simulink model "LQRPressureControl_simulation"  (R2020b)
settings: Solver=VariableStepAuto  StartTime=0.0  StopTime=36000  RelTol=1e-3
values from neighbouring files (symbols this model uses):
  A = double(A)    [ComponentUnitTests.m]    (also in ComponentUnitTests_linerization.m; InnerLoopNonLinSim.m; Kalman_filter_v2.m = [-0.3236   -0.0406   -0.1577   10.0671   -0.7623    0.0000)
  K = 5.4274    [Kalman_filter_final.m]
  ts = 0.025    [ComponentUnitTests.m]    (also in ComponentUnitTests_linerization.m; InnerLoopNonLinSim.m; Kalman_filter_final.m = 1; Kalman_filter_v2.m)
undefined symbols (not defined in the file or in its folder): Bp
libraries: TankPressure_Lib x1, VelocityDALQR_lib x1
settings Model: Creator=Christian  LastModifiedBy=Christian

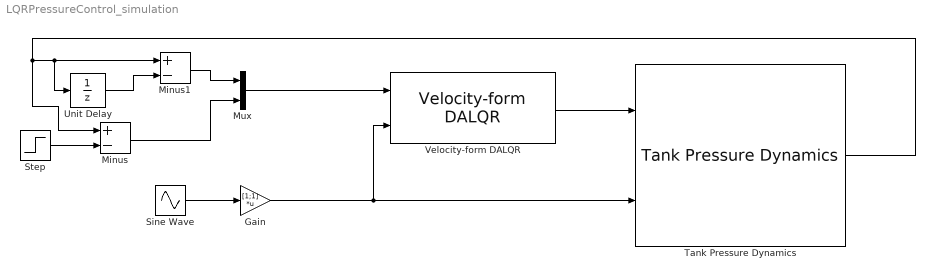
== system LQRPressureControl_simulation ==
  Gain : Gain  Gain=[1;1]  Multiplication=Matrix(K*u)
  Minus : Sum  Inputs=+-
  Minus1 : Sum  Inputs=+-
  Mux : Mux  Inputs=2
  Sine Wave : Sin  Amplitude=2  Bias=-2  Frequency=2*pi*1/3600  SampleTime=ts
  Step : Step  Time=3000  Before=2  After=5  SampleTime=0
  Tank Pressure Dynamics : TankPressure_Lib/Tank Pressure Dynamics  p_0=1  A=A  B_producer=Bp  B_consumer=Bc  Ts=ts
  Unit Delay : UnitDelay  InitialCondition=1  SampleTime=-1  HasFrameUpgradeWarning=on
  Velocity-form DALQR : VelocityDALQR_lib/Velocity-form DALQR  K=K  B_disturbance=Bc  B=Bp
  wires:
  Tank Pressure Dynamics/1 -> Minus/1, Unit Delay/1, Minus1/1
  Minus1/1 -> Mux/1
  Minus/1 -> Mux/2
  Step/1 -> Minus/2
  Gain/1 -> Tank Pressure Dynamics/2, Velocity-form DALQR/2
  Unit Delay/1 -> Minus1/2
  Mux/1 -> Velocity-form DALQR/1
  Velocity-form DALQR/1 -> Tank Pressure Dynamics/1
  Sine Wave/1 -> Gain/1
